simulink model "Cartesian_Regulation_ROS"  (R2022b)
settings: Solver=FixedStepAuto  StartTime=0.0  StopTime=inf  FixedStep=0.02  MaxStep=0.1  RelTol=1e-3
undefined symbols (not defined in the file): unicycle, X, x_f, Y, y_f
libraries: robotlib x3, simulink_extras x1, dspsigops x1
settings Model: Creator=hp 2021  LastModifiedBy=Musta
settings OptimizationCC: EnhancedBackFolding=on  PassReuseOutputArgsAs=Individual arguments  ZeroExternalMemoryAtStartup=off  ZeroInternalMemoryAtStartup=off  MaxStackSize=64  OptimizeBlockOrder=speed  DifferentSizesBufferReuse=on  OptimizationCustomize=off  EfficientTunableParamExpr=on
settings DebuggingCC: ParameterTunabilityLossMsg=error
settings HardwareCC: ProdBitPerPointer=32  ProdBitPerSizeT=32  ProdBitPerPtrDiffT=32  ProdLargestAtomicFloat=None  ProdIntDivRoundTo=Undefined  ProdEndianess=Unspecified  ProdWordSize=32  ProdHWDeviceType=Generic->Unspecified (assume 32-bit Generic)
settings ModelReferenceCC: EnableRefExpFcnMdlSchedulingChecks=on
settings SFSimCC: MATLABDynamicMemAlloc=off
settings RTWCC: Description=Embedded Coder  SystemTargetFile=ert.tlc  HardwareBoard=Robot Operating System (ROS)  TLCOptions="-aInlineSetEventsForThisBaseRateFcn=TLC_FALSE -aSuppressMultiTaskScheduler=TLC_FALSE  -aRateBasedStepFcn=0"  TemplateMakefile=ert_default_tmf  Toolchain=Catkin  TargetLang=C++
settings CodeAppCC: ForceParamTrailComments=on  IgnoreCustomStorageClasses=off  OperatorAnnotations=on  SimulinkDataObjDesc=on  SFDataObjDesc=on  InsertBlockDesc=on

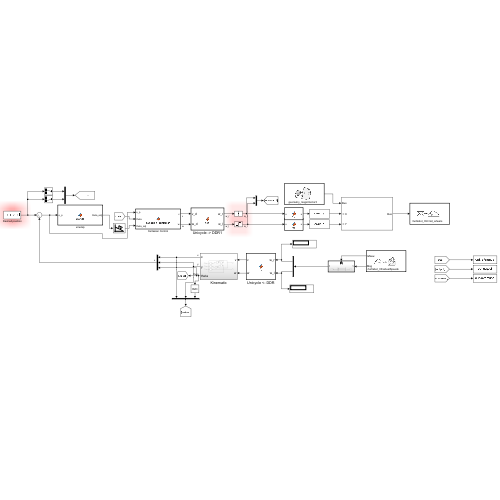
[thumbnail: Simulink's stored preview of the top-level diagram]
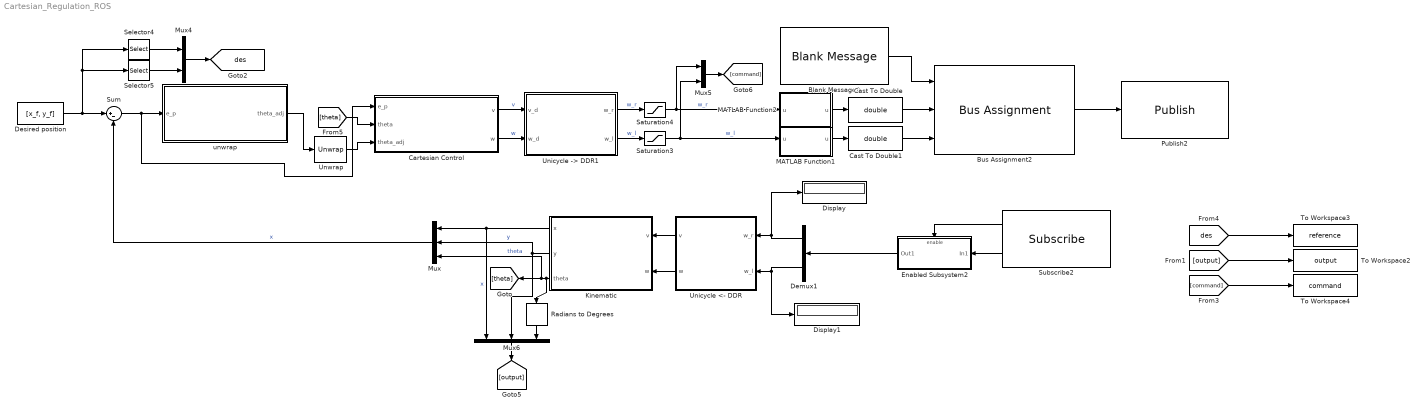
== system Cartesian_Regulation_ROS ==
  Blank Message2 : robotlib/Blank Message  messageClass=Message  entityType=geometry_msgs/Vector3  messageType=geometry_msgs/Vector3  SampleTime=0.02  legacyBusStruct=off
      settings: LibrarySourceBlock=roslib/ROS/Blank Message
  Bus Assignment2 : BusAssignment  AssignedSignals=X,Y
  Cartesian Control : MATLAB Function  TreatAsAtomicUnit=on
  Cast To Double : DataTypeConversion  OutDataTypeStr=double  SaturateOnIntegerOverflow=off  RndMeth=Floor
  Cast To Double1 : DataTypeConversion  OutDataTypeStr=double  SaturateOnIntegerOverflow=off  RndMeth=Floor
  Demux1 : Demux  Outputs=2
  Desired position : Constant  Value=[x_f, y_f]
  Display : Display
  Display1 : Display
  Enabled Subsystem2 : Subsystem  TreatAsAtomicUnit=on
  Kinematic : Subsystem
  MATLAB Function1 : MATLAB Function  TreatAsAtomicUnit=on
  MATLAB Function2 : MATLAB Function  TreatAsAtomicUnit=on
  Mux : Mux  Inputs=3
  Mux4 : Mux  Inputs=2
  Mux5 : Mux  Inputs=2
  Mux6 : Mux  Inputs=3
  Publish2 : robotlib/Publish  topicSource=Select from ROS network  topic=/turtlebot_03/cmd_wheels  messageType=geometry_msgs/Vector3  legacyBusStruct=off  messageQueueLength=1
      settings: LibrarySourceBlock=roslib/ROS/Publish
  Radians to Degrees : simulink_extras/Transformations/Radians to Degrees
  Saturation3 : Saturate  UpperLimit=unicycle.omegaWheelMax  LowerLimit=unicycle.omegaWheelMin
  Saturation4 : Saturate  UpperLimit=unicycle.omegaWheelMax  LowerLimit=unicycle.omegaWheelMin
  Selector4 : Selector  InputPortWidth=2  IndexOptions=Index vector (dialog)  Indices=1  OutputSizes=1
  Selector5 : Selector  InputPortWidth=2  IndexOptions=Index vector (dialog)  Indices=2  OutputSizes=1
  Subscribe2 : robotlib/Subscribe  topicSource=Select from ROS network  topic=/turtlebot_03/wheelSpeeds  messageType=geometry_msgs/Vector3  SampleTime=0.02  legacyBusStruct=off  messageQueueLength=1
      settings: LibrarySourceBlock=roslib/ROS/Subscribe
  Sum : Sum  Inputs=|+-
  To Workspace2 : ToWorkspace  VariableName=output  SaveFormat=Structure With Time  SampleTime=-1
  To Workspace3 : ToWorkspace  VariableName=reference  SaveFormat=Structure With Time  SampleTime=-1
  To Workspace4 : ToWorkspace  VariableName=command  SaveFormat=Structure With Time  SampleTime=-1
  "Unicycle -> DDR1" : MATLAB Function  TreatAsAtomicUnit=on
  Unicycle <- DDR : MATLAB Function  TreatAsAtomicUnit=on
  Unwrap : dspsigops/Unwrap  tol=0.99*pi  InputProcessing=Columns as channels (frame based)  running=off
  unwrap : MATLAB Function  TreatAsAtomicUnit=on
  tag scope: des=global
  wires:
  [command] -> To Workspace4/1
  [output] -> To Workspace2/1
  [des] -> To Workspace3/1
  Saturation4/1 -> MATLAB Function2/1("u "), Mux5/1  "w_r"
  Mux5/1 -> [command]
  Blank Message2/1 -> Bus Assignment2/1
  Bus Assignment2/1 -> Publish2/1
  "Unicycle -> DDR1"/2(w_l) -> Saturation3/1  "w_l"
  "Unicycle -> DDR1"/1(w_r) -> Saturation4/1  "w_r"
  Saturation3/1 -> MATLAB Function1/1("u "), Mux5/2  "w_l"
  Mux/1 -> Sum/2  "x"
  Subscribe2/2 -> Enabled Subsystem2/1(In1)
  Unicycle <- DDR/2(w) -> Kinematic/2(w)
  Demux1/2 -> Display1/1, Unicycle <- DDR/2(w_l)
  Kinematic/2(y) -> Mux/2, Mux6/2  "y"
  Kinematic/1(x) -> Mux/1, Mux6/1  "x"
  Unicycle <- DDR/1(v) -> Kinematic/1(v)
  Radians to Degrees/1 -> Mux6/3
  Kinematic/3(theta) -> Mux/3, [theta], Radians to Degrees/1  "theta"
  Demux1/1 -> Display/1, Unicycle <- DDR/1(w_r)
  Enabled Subsystem2/1(Out1) -> Demux1/1
  Mux6/1 -> [output]
  Subscribe2/1 -> Enabled Subsystem2/Enable
  MATLAB Function2/1(u) -> Cast To Double/1
  MATLAB Function1/1(u) -> Cast To Double1/1
  Cast To Double/1 -> Bus Assignment2/2
  Cast To Double1/1 -> Bus Assignment2/3
  Unwrap/1 -> Cartesian Control/3(theta_adj)
  Selector4/1 -> Mux4/1
  Sum/1 -> Cartesian Control/1(e_p), unwrap/1(e_p)
  [theta] -> Cartesian Control/2(theta)
  Mux4/1 -> [des]
  Desired position/1 -> Selector4/1, Selector5/1, Sum/1
  unwrap/1(theta_adj) -> Unwrap/1
  Selector5/1 -> Mux4/2
  Cartesian Control/1(v) -> "Unicycle -> DDR1"/1(v_d)  "v"
  Cartesian Control/2(w) -> "Unicycle -> DDR1"/2(w_d)  "w"

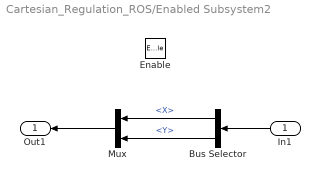
== system Cartesian_Regulation_ROS/Enabled Subsystem2 ==
  In1 : Inport
  Enable : EnablePort
  Bus Selector : BusSelector  OutputSignals=X,Y
  Mux : Mux  Inputs=2
  Out1 : Outport
  wires:
  Mux/1 -> Out1/1
  Bus Selector/1 -> Mux/1  "<X>"
  Bus Selector/2 -> Mux/2  "<Y>"
  In1/1 -> Bus Selector/1

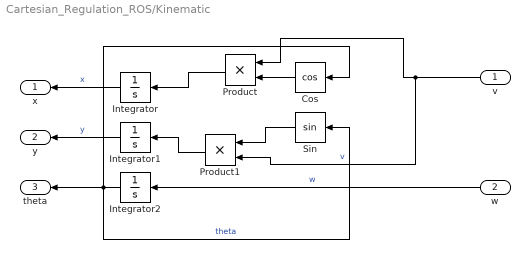
== system Cartesian_Regulation_ROS/Kinematic ==
  v : Inport
  w : Inport  Port=2
  Cos : Trigonometry  Operator=cos
  Integrator : Integrator  InitialCondition=unicycle.ic.x
  Integrator1 : Integrator  InitialCondition=unicycle.ic.y
  Integrator2 : Integrator  InitialCondition=unicycle.ic.theta
  Product : Product
  Product1 : Product
  Sin : Trigonometry
  x : Outport
  y : Outport  Port=2
  theta : Outport  Port=3
  wires:
  w/1 -> Integrator2/1  "w"
  Product/1 -> Integrator/1
  v/1 -> Product/1, Product1/2  "v"
  Cos/1 -> Product/2
  Integrator1/1 -> y/1  "y"
  Integrator/1 -> x/1  "x"
  Integrator2/1 -> theta/1, Sin/1, Cos/1  "theta"
  Product1/1 -> Integrator1/1
  Sin/1 -> Product1/1

== matlab function Cartesian_Regulation_ROS/unwrap ==
  data: theta_adj output; e_p input

function theta_adj = unwrap(e_p)

    theta_adj = mod(atan2(e_p(2),e_p(1)),2*pi);

end

== matlab function Cartesian_Regulation_ROS/Unicycle -> DDR1 ==
  data: v_d input; w_r output; w_d input; w_l output
function [w_r, w_l] = fcn(v_d, w_d)

    %#codegen
    coder.extrinsic('evalin')
    d = 0;                  % Needed in order to set variable class correctly
    r = 0;                  % Needed in order to set variable class correctly
    d = evalin('base','unicycle.d'); % Read value from workspace
    r = evalin('base','unicycle.r'); % Read value from workspace

    w_r = ((2 * v_d) + (w_d * d)) / (2 * r);
    w_l = ((2 * v_d) - (w_d * d)) / (2 * r);

end

== matlab function Cartesian_Regulation_ROS/MATLAB Function1 ==
  data: u input; u output
function u = fcn(u)


    if (isnan(u))
        u = 0.1;
    end

end

== matlab function Cartesian_Regulation_ROS/MATLAB Function2 ==
  data: u input; u output
function u = fcn(u)

    if (isnan(u))
        u = 0.1;
    end

end

== matlab function Cartesian_Regulation_ROS/Unicycle <- DDR ==
  data: w_r input; v output; w_l input; w output
function [v, w] = fcn(w_r, w_l)

    %#codegen
    coder.extrinsic('evalin')
    d = 0;                  % Needed in order to set variable class correctly
    r = 0;                  % Needed in order to set variable class correctly
    d = evalin('base','unicycle.d'); % Read value from workspace
    r = evalin('base','unicycle.r'); % Read value from workspace

    v = r*(w_r + w_l)/2; % rad/s
    w = r*(w_r - w_l)/d; % rad/s

end

== matlab function Cartesian_Regulation_ROS/Cartesian Control ==
  data: v output; w output; e_p input; theta input; theta_adj input
function [v,w] = cartesian_controller(e_p, theta, theta_adj)

    %#codegen
    coder.extrinsic('evalin')
    K_v = 0;                  % Needed in order to set variable class correctly
    K_w = 0;                  % Needed in order to set variable class correctly
    K_v = evalin('base','K_v'); % Read value from workspace
    K_w = evalin('base','K_w'); % Read value from workspace

    v = K_v * (e_p(1)*cos(theta) + e_p(2)*sin(theta));
    w = K_w * (theta_adj - theta);

end
